simulink model "schemat_lab6b"  (R2020a)
settings: Solver=VariableStepAuto  StartTime=0.0  StopTime=10.0  RelTol=1e-3
values from neighbouring files (symbols this model uses):
  A1 = 10    [gotowe2.m]    (also in lab7.m; lab8.m)
  a1 = 10    [gotowe2.m]    (also in lab7.m; lab8.m)
  a2 = 5    [gotowe2.m]    (also in lab7.m; lab8.m)
  A2 = 10    [gotowe2.m]    (also in lab7.m; lab8.m)
  dfwe1 = 0    [gotowe2.m]    (also in lab7.m; lab8.m = 0.5)
  dfwe2 = 0.1*fwemax    (= 0.5)    [gotowe2.m]    (also in lab7.m = 0; lab8.m = 0)
  fwe1 = 1    [gotowe2.m]    (also in lab7.m = mfwe1(i)*fwemax; lab8.m = mfwe1(i)*fwemax)
  fwe2 = mfwe2*fwemax    (= 2.5)    [gotowe2.m]    (also in lab7.m = 1; lab8.m = 1)
  h10 = (fwe1/a1)+h20    (= 0.8)    [gotowe2.m]    (also in lab7.m = 0.2; lab8.m = (fwe1/a1)+h20)
  h20 = (fwe1+fwe2)/(a2)    (= 0.7)    [gotowe2.m]    (also in lab7.m = 0.2; lab8.m = (fwe1+fwe2)/(a2))
settings Model: Creator=pc  LastModifiedBy=pc

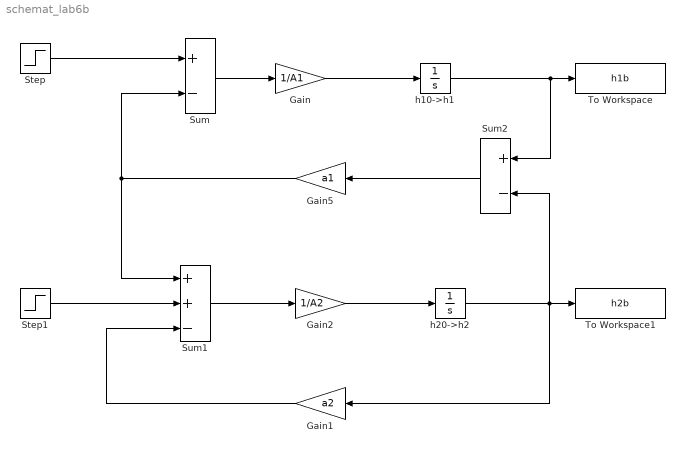
== system schemat_lab6b ==
  Gain : Gain  Gain=1/A1
  Gain1 : Gain  Gain=a2
  Gain2 : Gain  Gain=1/A2
  Gain5 : Gain  Gain=a1
  Step : Step  Time=5  Before=fwe1  After=fwe1+dfwe1  SampleTime=0
  Step1 : Step  Time=5  Before=fwe2  After=fwe2+dfwe2  SampleTime=0
  Sum : Sum  Inputs=+-
  Sum1 : Sum  Inputs=++-
  Sum2 : Sum  Inputs=+-
  To Workspace : ToWorkspace  VariableName=h1b  SampleTime=-1
  To Workspace1 : ToWorkspace  VariableName=h2b  SampleTime=-1
  h10->h1 : Integrator  InitialCondition=h10
  h20->h2 : Integrator  InitialCondition=h20
  wires:
  Sum/1 -> Gain/1
  Gain2/1 -> h20->h2/1
  Gain5/1 -> Sum/2, Sum1/1
  Gain1/1 -> Sum1/3
  h20->h2/1 -> Gain1/1, Sum2/2, To Workspace1/1
  Gain/1 -> h10->h1/1
  Step1/1 -> Sum1/2
  Sum1/1 -> Gain2/1
  Sum2/1 -> Gain5/1
  h10->h1/1 -> Sum2/1, To Workspace/1
  Step/1 -> Sum/1
